simulink model "vafid_closed_loop_validation"  (R2026a)
settings: Solver=FixedStepDiscrete  StopTime=6  FixedStep=5e-5
undefined symbols (not defined in the file or in its folder): vafid_validation_model_data
settings Model: Creator=ASUS  LastModifiedBy=ASUS

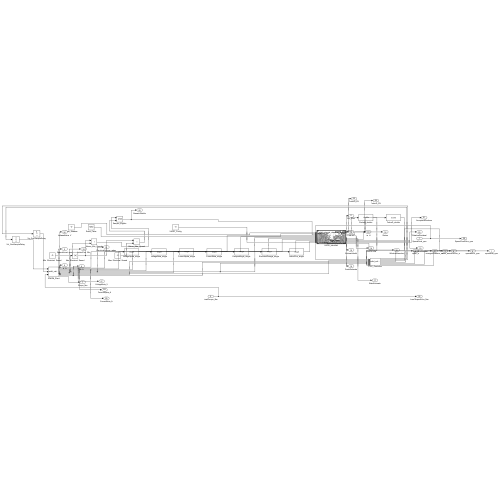
[thumbnail: Simulink's stored preview of the top-level diagram]
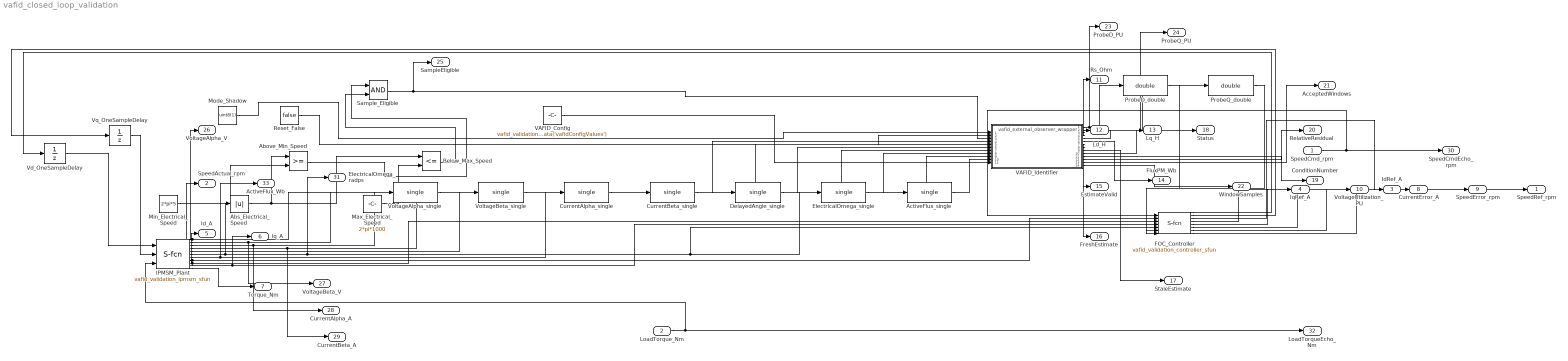
== system vafid_closed_loop_validation ==
  SpeedCmd_rpm : Inport
  LoadTorque_Nm : Inport  Port=2
  Above_Min_Speed : RelationalOperator  OutDataTypeStr=boolean  RndMeth=Simplest  InputSameDT=off
  Abs_Electrical_Speed : Abs  SaturateOnIntegerOverflow=off
  ActiveFlux_single : DataTypeConversion  OutDataTypeStr=single  SaturateOnIntegerOverflow=off  RndMeth=Floor
  Below_Max_Speed : RelationalOperator  Operator=<=  OutDataTypeStr=boolean  RndMeth=Simplest  InputSameDT=off
  CurrentAlpha_single : DataTypeConversion  OutDataTypeStr=single  SaturateOnIntegerOverflow=off  RndMeth=Floor
  CurrentBeta_single : DataTypeConversion  OutDataTypeStr=single  SaturateOnIntegerOverflow=off  RndMeth=Floor
  DelayedAngle_single : DataTypeConversion  OutDataTypeStr=single  SaturateOnIntegerOverflow=off  RndMeth=Floor
  ElectricalOmega_single : DataTypeConversion  OutDataTypeStr=single  SaturateOnIntegerOverflow=off  RndMeth=Floor
  FOC_Controller : M-S-Function  FunctionName=vafid_validation_controller_sfun  Parameters=vafid_validation_model_data('controller')
  IPMSM_Plant : M-S-Function  FunctionName=vafid_validation_ipmsm_sfun  Parameters=vafid_validation_model_data('plant')
  Max_Electrical_Speed : Constant  Value=2*pi*1000
  Min_Electrical_Speed : Constant  Value=2*pi*5
  Mode_Shadow : Constant  Value=uint8(1)  OutDataTypeStr=uint8
  ProbeD_double : DataTypeConversion  OutDataTypeStr=double  SaturateOnIntegerOverflow=off  RndMeth=Floor
  ProbeQ_double : DataTypeConversion  OutDataTypeStr=double  SaturateOnIntegerOverflow=off  RndMeth=Floor
  Reset_False : Constant  Value=false  OutDataTypeStr=boolean
  Sample_Eligible : Logic  AllPortsSameDT=off  OutDataTypeStr=boolean
  VAFID_Config : Constant  Value=vafid_validation_model_data('vafidConfigValues')  OutDataTypeStr=single
  VAFID_Identifier : ModelReference  ModelNameDialog=vafid_external_observer_wrapper  SimulationMode=Normal  ModelReferenceVersion=1.2
  Vd_OneSampleDelay : UnitDelay  SampleTime=5e-5
  VoltageAlpha_single : DataTypeConversion  OutDataTypeStr=single  SaturateOnIntegerOverflow=off  RndMeth=Floor
  VoltageBeta_single : DataTypeConversion  OutDataTypeStr=single  SaturateOnIntegerOverflow=off  RndMeth=Floor
  Vq_OneSampleDelay : UnitDelay  SampleTime=5e-5
  SpeedRef_rpm : Outport
  SpeedActual_rpm : Outport  Port=2
  IdRef_A : Outport  Port=3
  IqRef_A : Outport  Port=4
  Id_A : Outport  Port=5
  Iq_A : Outport  Port=6
  Torque_Nm : Outport  Port=7
  CurrentError_A : Outport  Port=8
  SpeedError_rpm : Outport  Port=9
  VoltageUtilization_PU : Outport  Port=10
  Rs_Ohm : Outport  Port=11
  Ld_H : Outport  Port=12
  Lq_H : Outport  Port=13
  FluxPM_Wb : Outport  Port=14
  EstimateValid : Outport  Port=15
  FreshEstimate : Outport  Port=16
  StaleEstimate : Outport  Port=17
  Status : Outport  Port=18
  ConditionNumber : Outport  Port=19
  RelativeResidual : Outport  Port=20
  AcceptedWindows : Outport  Port=21
  WindowSamples : Outport  Port=22
  ProbeD_PU : Outport  Port=23
  ProbeQ_PU : Outport  Port=24
  SampleEligible : Outport  Port=25
  VoltageAlpha_V : Outport  Port=26
  VoltageBeta_V : Outport  Port=27
  CurrentAlpha_A : Outport  Port=28
  CurrentBeta_A : Outport  Port=29
  SpeedCmdEcho_rpm : Outport  Port=30
  ElectricalOmega_radps : Outport  Port=31
  LoadTorqueEcho_Nm : Outport  Port=32
  ActiveFlux_Wb : Outport  Port=33
  wires:
  Max_Electrical_Speed/1 -> Below_Max_Speed/2
  Min_Electrical_Speed/1 -> Above_Min_Speed/2
  Abs_Electrical_Speed/1 -> Below_Max_Speed/1, Above_Min_Speed/1
  Vd_OneSampleDelay/1 -> IPMSM_Plant/1
  Vq_OneSampleDelay/1 -> IPMSM_Plant/2
  ActiveFlux_single/1 -> VAFID_Identifier/10
  ElectricalOmega_single/1 -> VAFID_Identifier/9
  DelayedAngle_single/1 -> VAFID_Identifier/8
  IPMSM_Plant/5 -> DelayedAngle_single/1
  CurrentBeta_single/1 -> VAFID_Identifier/7
  CurrentAlpha_single/1 -> VAFID_Identifier/6
  VoltageBeta_single/1 -> VAFID_Identifier/5
  VoltageAlpha_single/1 -> VAFID_Identifier/4
  Mode_Shadow/1 -> VAFID_Identifier/1
  Reset_False/1 -> VAFID_Identifier/2
  VAFID_Config/1 -> VAFID_Identifier/11
  VAFID_Identifier/14 -> WindowSamples/1
  VAFID_Identifier/10 -> Status/1
  VAFID_Identifier/9 -> StaleEstimate/1
  VAFID_Identifier/8 -> FreshEstimate/1
  VAFID_Identifier/7 -> EstimateValid/1
  VAFID_Identifier/6 -> FluxPM_Wb/1
  VAFID_Identifier/5 -> Lq_H/1
  VAFID_Identifier/4 -> Ld_H/1
  VAFID_Identifier/3 -> Rs_Ohm/1
  FOC_Controller/5 -> VoltageUtilization_PU/1
  FOC_Controller/7 -> SpeedError_rpm/1
  FOC_Controller/6 -> CurrentError_A/1
  IPMSM_Plant/11 -> Torque_Nm/1
  FOC_Controller/4 -> IqRef_A/1
  FOC_Controller/8 -> SpeedRef_rpm/1
  Sample_Eligible/1 -> VAFID_Identifier/3, SampleEligible/1
  IPMSM_Plant/6 -> FOC_Controller/5, ElectricalOmega_single/1, ElectricalOmega_radps/1, Abs_Electrical_Speed/1
  IPMSM_Plant/1 -> VoltageAlpha_single/1, VoltageAlpha_V/1
  IPMSM_Plant/2 -> VoltageBeta_single/1, VoltageBeta_V/1
  IPMSM_Plant/3 -> CurrentAlpha_single/1, CurrentAlpha_A/1
  IPMSM_Plant/4 -> CurrentBeta_single/1, CurrentBeta_A/1
  IPMSM_Plant/7 -> ActiveFlux_single/1, ActiveFlux_Wb/1
  VAFID_Identifier/1 -> ProbeD_double/1, ProbeD_PU/1
  ProbeD_double/1 -> FOC_Controller/6
  VAFID_Identifier/2 -> ProbeQ_double/1, ProbeQ_PU/1
  ProbeQ_double/1 -> FOC_Controller/7
  IPMSM_Plant/10 -> FOC_Controller/4, Iq_A/1
  IPMSM_Plant/9 -> FOC_Controller/3, Id_A/1
  IPMSM_Plant/8 -> FOC_Controller/2, SpeedActual_rpm/1
  FOC_Controller/1 -> Vd_OneSampleDelay/1
  FOC_Controller/2 -> Vq_OneSampleDelay/1
  Above_Min_Speed/1 -> Sample_Eligible/1
  Below_Max_Speed/1 -> Sample_Eligible/2
  LoadTorque_Nm/1 -> IPMSM_Plant/3, LoadTorqueEcho_Nm/1
  SpeedCmd_rpm/1 -> SpeedCmdEcho_rpm/1, FOC_Controller/1
  FOC_Controller/3 -> IdRef_A/1
  VAFID_Identifier/11 -> ConditionNumber/1
  VAFID_Identifier/12 -> RelativeResidual/1
  VAFID_Identifier/13 -> AcceptedWindows/1
